simulink model "Afr"  (R2021a)
settings: Solver=ode45  StartTime=0.0  StopTime=10.0  RelTol=1e-3  EnableMultiTasking=on
undefined symbols (not defined in the file): Afr_facLambdaReqMan, Afr_facRatioMan, Afr_facStoich, Afr_flgLambdaReqOverride, Afr_flgRatioOverride
libraries: simulink x1
settings Model: Creator=YAL9FE  LastModifiedBy=FPR9FE
settings SolverCC: AlgebraicLoopSolver=TrustRegion
settings DataIOCC: LimitDataPoints=on  SaveFormat=Array  SignalLoggingSaveFormat=ModelDataLogs  ReturnWorkspaceOutputs=off
settings OptimizationCC: ExpressionDepthLimit=2147483647  LifeSpan=inf
settings DebuggingCC: UnderspecifiedInitializationDetection=Classic  MergeDetectMultiDrivingBlocksExec=none  SolverPrmCheckMsg=warning  FcnCallInpInsideContextMsg=warning  StateNameClashWarn=warning  SFUnexpectedBacktrackingDiag=warning  SFNoUnconditionalDefaultTransitionDiag=warning  SFExecutionAtInitializationDiag=none  SFMachineParentedDataDiag=warning  ArithmeticOperatorsInVariantConditions=warning
settings HardwareCC: ProdBitPerPointer=32  ProdBitPerSizeT=32  ProdBitPerPtrDiffT=32  ProdLargestAtomicFloat=None  ProdIntDivRoundTo=Undefined  ProdEndianess=Unspecified  ProdWordSize=32  ProdHWDeviceType=32-bit Generic
settings ModelReferenceCC: PropagateSignalLabelsOutOfModel=off
settings SFSimCC: SimUseLocalCustomCode=off  CustomCodeUndefinedFunction=UseInterfaceOnly
settings RTWCC: RTWUseLocalCustomCode=off
settings CodeAppCC: StateflowObjectComments=on
settings GRTTargetCC: TargetLangStandard=C89/C90 (ANSI)  CombineOutputUpdateFcns=off  GRTInterface=on
settings ConfigComp: CovMetricSettings=dw  CovSaveCumulativeToWorkspaceVar=on  CovSaveSingleToWorkspaceVar=on  CovExternalEMLEnable=off  CovSFcnEnable=off

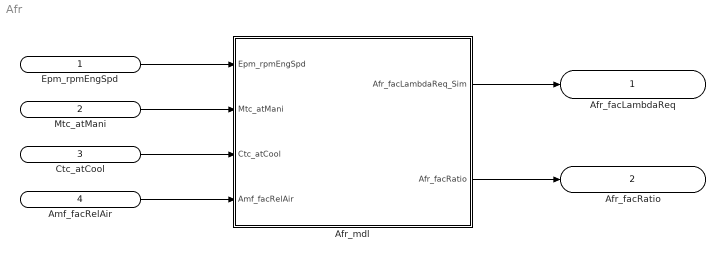
== system Afr ==
  Epm_rpmEngSpd : Inport
  Mtc_atMani : Inport  Port=2
  Ctc_atCool : Inport  Port=3
  Amf_facRelAir : Inport  Port=4
  Afr_mdl : Subsystem  mask(Functions){}
      mask help: AirFuelRatio
      mask Display:
      | image(imread('AirFuelRatio.jpg'))
      | port_label('input',1,'Epm_rpmEngSpd_Sim')
      | port_label('input',2,'Mtc_atMani_Sim')
      | port_label('input',3,'Ctc_atCool_Sim')
      | port_label('input',4,'Amf_facRelAir_Sim')
      | port_label('output',1,'Afr_facLambdaReq_Sim')
      | port_label('output',2,'Afr_facRatio_Sim')
  Afr_facLambdaReq : Outport
  Afr_facRatio : Outport  Port=2
  wires:
  Epm_rpmEngSpd/1 -> Afr_mdl/1(Epm_rpmEngSpd)
  Mtc_atMani/1 -> Afr_mdl/2(Mtc_atMani)
  Ctc_atCool/1 -> Afr_mdl/3(Ctc_atCool)
  Amf_facRelAir/1 -> Afr_mdl/4(Amf_facRelAir)
  Afr_mdl/1(Afr_facLambdaReq_Sim) -> Afr_facLambdaReq/1
  Afr_mdl/2(Afr_facRatio) -> Afr_facRatio/1

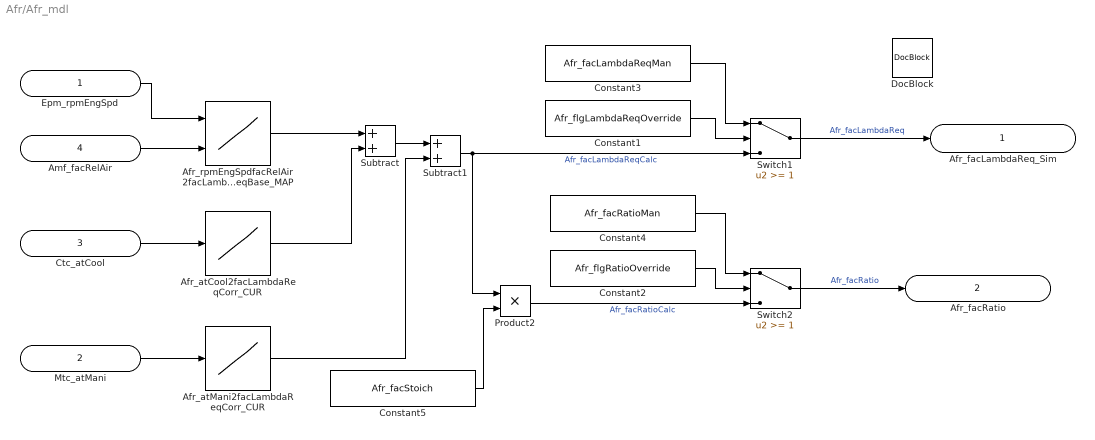
== system Afr/Afr_mdl ==
  Epm_rpmEngSpd : Inport
  Mtc_atMani : Inport  Port=2
  Ctc_atCool : Inport  Port=3
  Amf_facRelAir : Inport  Port=4
  Afr_atCool2facLambdaReqCorr_CUR : Lookup_n-D  NumberOfTableDimensions=1  BreakpointsForDimension1=[1:3]  Table=[4 5 6]  ExtrapMethod=Clip  InputSameDT=on
  Afr_atMani2facLambdaReqCorr_CUR : Lookup_n-D  NumberOfTableDimensions=1  BreakpointsForDimension1=[1:3]  Table=[4 5 6]  ExtrapMethod=Clip  InputSameDT=on
  Afr_rpmEngSpdfacRelAir2facLambdaReqBase_MAP : Lookup_n-D  BreakpointsForDimension1=[1:3]  BreakpointsForDimension2=[1:3]  ExtrapMethod=Clip  InputSameDT=on
      settings: InputPortMap=u0,u1
  Constant1 : Constant  Value=Afr_flgLambdaReqOverride
  Constant2 : Constant  Value=Afr_flgRatioOverride
  Constant3 : Constant  Value=Afr_facLambdaReqMan
  Constant4 : Constant  Value=Afr_facRatioMan
  Constant5 : Constant  Value=Afr_facStoich
  DocBlock : simulink/Model-Wide Utilities/DocBlock  DocumentType=Text
      content=|
      | In the air-fuel ratio (AirFuelRatio) module, the required air-to-fuel ratio is calculated on the basis of a specified lambda value. For this purpose, a base value for lambda is determined via the map Afr_rpmEngSpdfacRelAir2facLambdaReqBase_MAP from the speed Epm_rpmEngSpd and the relative filling Amf_facRelAir and then corrected. Based on experience, the basic parameterization is here across all speed ranges in the partial load range, i. H. at relative fillings below 80%, at λ= 1.0 and in the full load range over 120% at λ= 0.7. A linear interpolation takes place in the transition area in between.
      |
      | On the one hand, corrections are made depending on the coolant temperature Ctc_atCool, which is calculated using the characteristic curve Afr_atCool2facLambdaReqCorr_CUR. When the engine is cold, the mixture is enriched to warm up the engine, which becomes zero from around 50°C. On the other hand, a fresh air temperature-dependent (Mtc_atMani via Afr_atMani2facLambdaReqCorr_CUR ) enrichment or leaning can be carried out. This map is set to zero from the start. The lambda value calculated in this way can be manually overwritten with Afr_facLambdaReqMan by setting the flag Afr_flgLambdaReqOverride before it is exported as a message. Equation 5.7 shows the calculations for the lambda value.
      |
      | Furthermore, the air-fuel ratio Afr_facRatio is calculated from the lambda value by multiplying it with the stoichiometric factor Afr_facStoich Equation 5.8. Here, too, there is the option of manually overwriting the calculated value with Afr_facRatioMan (setting the Afr_flgRatioOverride flag) before it is exported as a message. The Afr_calc function is evaluated in the synchronous grid.
  Product2 : Product  OutDataTypeStr=Inherit: Same as first input
  Subtract : Sum  OutDataTypeStr=Inherit: Same as first input
  Subtract1 : Sum  OutDataTypeStr=Inherit: Same as first input
  Switch1 : Switch  Threshold=1
  Switch2 : Switch  Threshold=1
  Afr_facLambdaReq_Sim : Outport
  Afr_facRatio : Outport  Port=2
  wires:
  Epm_rpmEngSpd/1 -> Afr_rpmEngSpdfacRelAir2facLambdaReqBase_MAP/1
  Amf_facRelAir/1 -> Afr_rpmEngSpdfacRelAir2facLambdaReqBase_MAP/2
  Afr_rpmEngSpdfacRelAir2facLambdaReqBase_MAP/1 -> Subtract/1
  Subtract/1 -> Subtract1/1
  Ctc_atCool/1 -> Afr_atCool2facLambdaReqCorr_CUR/1
  Afr_atCool2facLambdaReqCorr_CUR/1 -> Subtract/2
  Mtc_atMani/1 -> Afr_atMani2facLambdaReqCorr_CUR/1
  Afr_atMani2facLambdaReqCorr_CUR/1 -> Subtract1/2
  Subtract1/1 -> Switch1/3, Product2/1  "Afr_facLambdaReqCalc"
  Constant1/1 -> Switch1/2
  Constant3/1 -> Switch1/1
  Switch1/1 -> Afr_facLambdaReq_Sim/1  "Afr_facLambdaReq"
  Switch2/1 -> Afr_facRatio/1  "Afr_facRatio"
  Product2/1 -> Switch2/3  "Afr_facRatioCalc"
  Constant5/1 -> Product2/2
  Constant2/1 -> Switch2/2
  Constant4/1 -> Switch2/1
